simulink model "Simulink_practice2"  (R2021b)
settings: Solver=ode4  StartTime=0.0  StopTime=TIME.Final  FixedStep=TIME.Ts  RelTol=1e-3
values from neighbouring files (symbols this model uses):
  K1 = 1.    (= 1)    [simulink_simulation.m]
  K2 = 0.6    [simulink_simulation.m]
  K3 = 0.05    [simulink_simulation.m]
  K4 = 1.5    [simulink_simulation.m]
  TIME = struct('Ts'   , 1e-3,                'Start', 0.0 ,                'Final',20.0 ,                'stage', 0.15,                'time' , 0   ,                'Ntime', 0   )    [UAV_simulation.m]    (also in main_simulink_practice.m = struct('Start', 0.0,                'Ts'   , 1e-3,          ; main_untitled1.m = struct('Ts', 1e-3,                'Final',30,               ; main_untitled2.m = struct('Ts', 1e-3,                'Start', 0.0,             ; script_simulation.m = struct('Start', 0.0  ,                'Final',30.0  ,       )
settings Model: Creator=jinkwak  LastModifiedBy=jinkwak

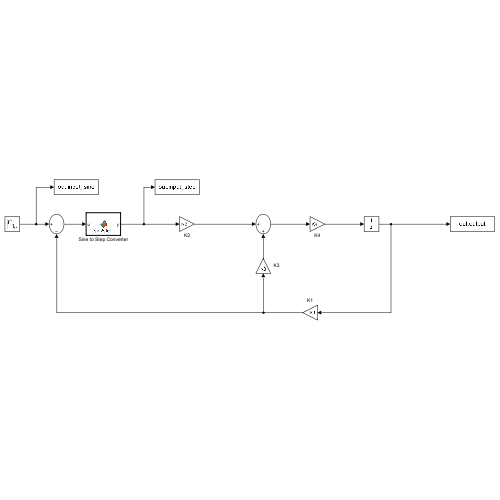
[thumbnail: Simulink's stored preview of the top-level diagram]
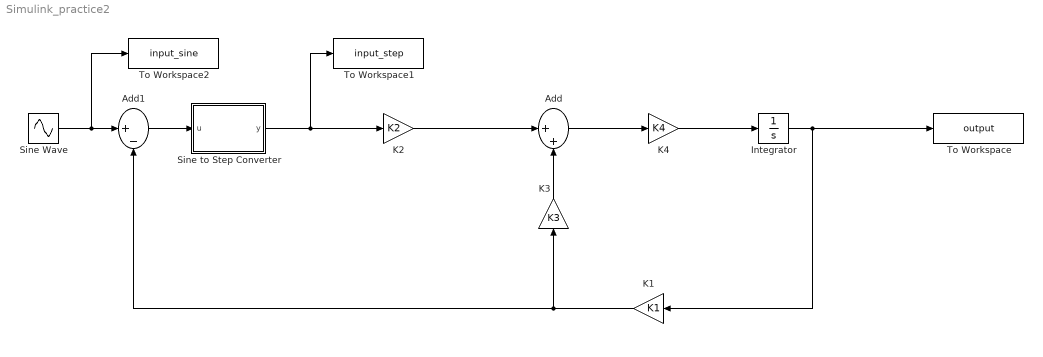
== system Simulink_practice2 ==
  Add : Sum  Inputs=|++
  Add1 : Sum  Inputs=|+-
  Integrator : Integrator
  K1 : Gain  Gain=K1
  K2 : Gain  Gain=K2
  K3 : Gain  Gain=K3
  K4 : Gain  Gain=K4
  Sine Wave : Sin  SampleTime=TIME.Ts
  Sine to Step Converter : MATLAB Function  TreatAsAtomicUnit=on
  To Workspace : ToWorkspace  VariableName=output  SampleTime=TIME.Ts
      settings: Save2DSignal=2-D array (concatenate along first dimension)
  To Workspace1 : ToWorkspace  VariableName=input_step  SampleTime=TIME.Ts
      settings: Save2DSignal=2-D array (concatenate along first dimension)
  To Workspace2 : ToWorkspace  VariableName=input_sine  SampleTime=TIME.Ts
      settings: Save2DSignal=2-D array (concatenate along first dimension)
  wires:
  K2/1 -> Add/1
  K3/1 -> Add/2
  Add/1 -> K4/1
  K4/1 -> Integrator/1
  Integrator/1 -> To Workspace/1, K1/1
  K1/1 -> Add1/2, K3/1
  Sine to Step Converter/1(y) -> To Workspace1/1, K2/1
  Add1/1 -> Sine to Step Converter/1(u)
  Sine Wave/1 -> To Workspace2/1, Add1/1

== matlab function Simulink_practice2/Sine to Step Converter ==
  data: u input; y output
function y = sin2step(u)
if u< 0
    y = -1;
else
    y = 1;
end
